simulink model "StateEstimatorForActuatorDelay"  (R2020b)
settings: Solver=FixedStepAuto  StartTime=0.0  StopTime=.5  RelTol=1e-3
values from neighbouring files (symbols this model uses):
  F = eye(6)    [MEKFAttitudeOnly.m]
  Moments = [0; 0; 0]    [Forces_and_Moments_Calculator.m]
  q = x(13:16)    [AdaptiveLQR.m]    (also in MEKF.m = nominal_state(4:7); MEKFAttitudeOnly.m = [1 0 0 0]; MEKF_old.m = nominal_state(4:7); NonlinearStateEstimationForActuatorDelay.m = x(4:7))
  r = sym('r', [3 1])    [StateSpaceController.m]    (also in TimeDelayCompensationElevator.m = [0;0]; Tracker.m = [0; 0; -(rocket_length - Average_cg)])
  ThrustTable = xlsread('F15_Thrust','Sheet1')    [ImpactVelocityNotParallelMatlab.m]    (also in OneDLanding.m; ParallelImpactVelocity.m; RunImpactVelocityParforCompiled.m)
undefined symbols (not defined in the file or in its folder): Earth, HeightAboveSeaLevel, initial_q, initial_qi, initial_w, Light, masscgI, MIL, t0, WGS84
libraries: shared6dof x4, aerolibwind2 x3, vrlib x2, shared6dofsys x2, sharedtransform x2, aerolibbdyn x1, aerolibtransform2 x1, simulink x1, sharedutil x1
settings Model: SimulationMode=accelerator  Creator=rag  LastModifiedBy=rag
settings DataIOCC: SaveFinalState=on  SaveOutput=off  SignalLogging=off  DSMLogging=off  SaveTime=off
settings OptimizationCC: DefaultParameterBehavior=Inlined  UseDivisionForNetSlopeComputation=on  GainParamInheritBuiltInType=on  UseFloatMulNetSlope=on  InlineInvariantSignals=on  EfficientFloat2IntCast=on  LifeSpan=1
settings HardwareCC: ProdLongLongMode=on
settings SFSimCC: MATLABDynamicMemAlloc=off
settings RTWCC: GenerateReport=on  LaunchReport=on
settings CodeAppCC: ForceParamTrailComments=on
settings GRTTargetCC: CombineSignalStateStructs=on  MatFileLogging=off  SupportVariableSizeSignals=on

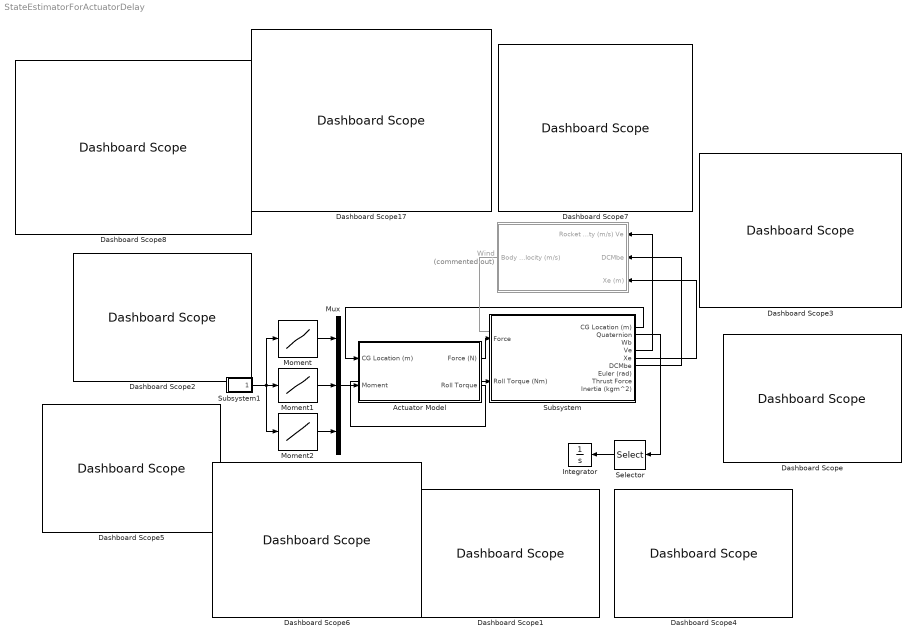
== system StateEstimatorForActuatorDelay ==
  Actuator Model : Subsystem
  Dashboard Scope{,1..8,17} (10 alike) : DashboardScope
  Integrator : Integrator  InitialCondition=initial_qi
  Moment : Lookup_n-D  NumberOfTableDimensions=1  BreakpointsForDimension1=Moments(:,1)  BreakpointsForDimension2=Moments(:,1)  BreakpointsForDimension3=Moments(:,1)  BreakpointsForDimension1FirstPoint=0  BreakpointsForDimension1Spacing=1.5e-5  Table=Moments(:,2)  ExtrapMethod=Clip  InternalRulePriority=Speed  RndMeth=Simplest  InputSameDT=on
  Moment1 : Lookup_n-D  NumberOfTableDimensions=1  BreakpointsForDimension1=Moments(:,1)  BreakpointsForDimension2=Moments(:,1)  BreakpointsForDimension3=Moments(:,1)  BreakpointsForDimension1FirstPoint=0  BreakpointsForDimension1Spacing=1.5e-5  Table=Moments(:,3)  ExtrapMethod=Clip  InternalRulePriority=Speed  RndMeth=Simplest  InputSameDT=on
  Moment2 : Lookup_n-D  NumberOfTableDimensions=1  BreakpointsForDimension1=Moments(:,1)  BreakpointsForDimension2=Moments(:,1)  BreakpointsForDimension3=Moments(:,1)  BreakpointsForDimension1FirstPoint=0  BreakpointsForDimension1Spacing=1.5e-5  Table=Moments(:,4)  ExtrapMethod=Clip  InternalRulePriority=Speed  RndMeth=Simplest  InputSameDT=on
  Mux : Mux  Inputs=3
  Selector : Selector  InputPortWidth=4  IndexOptions=Index vector (dialog)  Indices=[2:4]  OutputSizes=1
  Subsystem : Subsystem
  Subsystem1 : Subsystem
  Wind : Subsystem  Commented=on
  wires:
  Subsystem/1(CG Location (m)) -> Actuator Model/1(CG Location (m))
  Wind/1(Body Wind Velocity (m/s)) -> ?
  Actuator Model/1(Force (N)) -> Subsystem/1(Force)
  Actuator Model/2(Roll Torque) -> Subsystem/2(Roll Torque (Nm))
  Subsystem/4(Ve) -> Wind/1(Rocket velocity (m/s) Ve)
  Subsystem/6(DCMbe) -> Wind/2(DCMbe)
  Subsystem/5(Xe) -> Wind/3(Xe (m))
  Selector/1 -> Integrator/1
  Subsystem/2(Quaternion) -> Selector/1
  Moment/1 -> Mux/1
  Mux/1 -> Actuator Model/2(Moment)
  Moment1/1 -> Mux/2
  Moment2/1 -> Mux/3
  Subsystem1/1(time) -> Moment2/1, Moment/1, Moment1/1

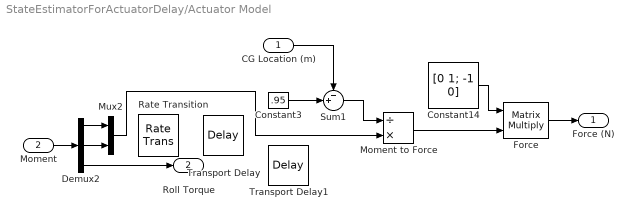
== system StateEstimatorForActuatorDelay/Actuator Model ==
  CG Location (m) : Inport
  Moment : Inport  Port=2
  Constant14 : Constant  Value=[0 1; -1 0]
  Constant3 : Constant  Value=.95
  Demux2 : Demux  Outputs=3
  Force : Product  Multiplication=Matrix(*)
  Moment to Force : Product  Inputs=/*
  Mux2 : Mux  Inputs=2
  Rate Transition : RateTransition  OutPortSampleTime=0.02
  Sum1 : Sum  Inputs=-+|
  Transport Delay : TransportDelay  DelayTime=0.07  TransDelayFeedthrough=on
  Transport Delay1 : TransportDelay  DelayTime=0.01  TransDelayFeedthrough=on
  Force (N) : Outport
  Roll Torque : Outport  Port=2
  wires:
  Demux2/1 -> Mux2/1
  Mux2/1 -> Moment to Force/2
  Sum1/1 -> Moment to Force/1
  Moment to Force/1 -> Force/2
  Constant3/1 -> Sum1/2
  Demux2/2 -> Mux2/2
  Moment/1 -> Demux2/1
  Constant14/1 -> Force/1
  Demux2/3 -> Roll Torque/1
  CG Location (m)/1 -> Sum1/1
  Force/1 -> Force (N)/1

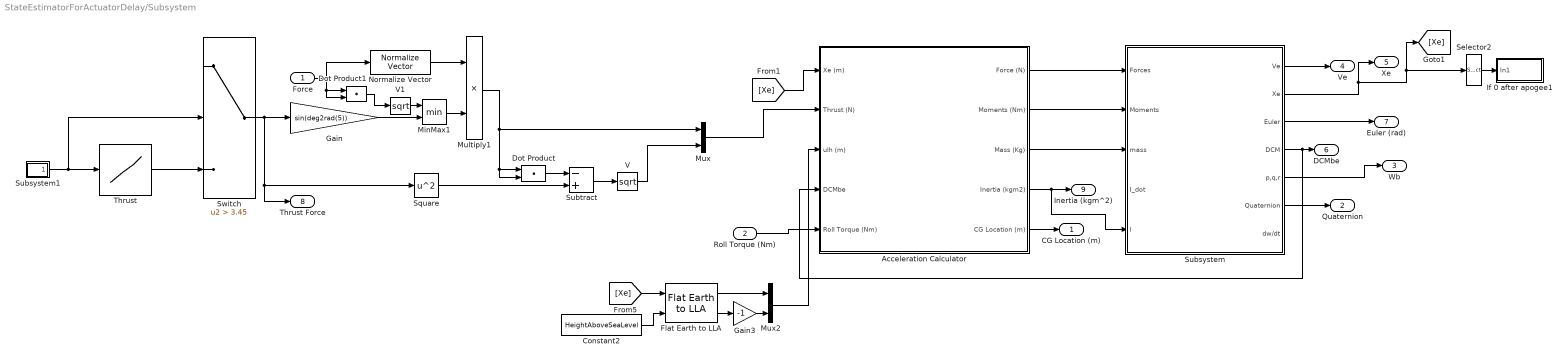
== system StateEstimatorForActuatorDelay/Subsystem ==
  Force : Inport  PortDimensions=2
  Roll Torque (Nm) : Inport  Port=2
  Acceleration Calculator : Subsystem
  Constant2 : Constant  Value=HeightAboveSeaLevel
  Dot Product : DotProduct  SaturateOnIntegerOverflow=on  OutDataTypeStr=Inherit: Inherit via internal rule
  Dot Product1 : DotProduct  SaturateOnIntegerOverflow=on  OutDataTypeStr=Inherit: Inherit via internal rule
  Flat Earth to LLA : aerolibtransform2/Flat Earth to LLA  units=Metric (MKS)  ptype=Earth (WGS84)  F=1/298.257223563  R=6378137  refPosPort=off  LL0=[21.318358277648 -157.9232805920725]  psi=0
  Gain : Gain  Gain=sin(deg2rad(5))
  Gain3 : Gain  Gain=-1
  If 0 after apogee1 : Subsystem
  MinMax1 : MinMax  Inputs=2
  Multiply1 : Product  Inputs=**
  Mux : Mux  Inputs=2
  Mux2 : Mux  Inputs=2
  Normalize Vector : vrlib/Utilities/Normalize Vector  maxzero=0
  Selector2 : Selector  InputPortWidth=3  IndexOptions=Index vector (dialog)  Indices=[3]  OutputSizes=1
  Square : Math  Operator=square  SignedPower=on  SaturateOnIntegerOverflow=on
  Subsystem : Subsystem
  Subsystem1 : Subsystem
  Subtract : Sum  Inputs=-+
  Switch : Switch  Criteria=u2 > Threshold  Threshold=3.45
  Thrust : Lookup_n-D  NumberOfTableDimensions=1  BreakpointsForDimension1=ThrustTable(:,1)  BreakpointsForDimension1FirstPoint=0  BreakpointsForDimension1Spacing=1.5e-5  Table=ThrustTable(:,2)  ExtrapMethod=Clip  InternalRulePriority=Speed  RndMeth=Simplest  InputSameDT=on
  V : Math  Operator=sqrt  SignedPower=on  SaturateOnIntegerOverflow=on
  V1 : Math  Operator=sqrt  SignedPower=on  SaturateOnIntegerOverflow=on
  CG Location (m) : Outport  VectorParamsAs1DForOutWhenUnconnected=off
  Quaternion : Outport  Port=2  VectorParamsAs1DForOutWhenUnconnected=off
  Wb : Outport  Port=3  VectorParamsAs1DForOutWhenUnconnected=off
  Ve : Outport  Port=4  VectorParamsAs1DForOutWhenUnconnected=off
  Xe : Outport  Port=5  VectorParamsAs1DForOutWhenUnconnected=off
  DCMbe : Outport  Port=6  VectorParamsAs1DForOutWhenUnconnected=off
  Euler (rad) : Outport  Port=7  VectorParamsAs1DForOutWhenUnconnected=off
  Thrust Force : Outport  Port=8  VectorParamsAs1DForOutWhenUnconnected=off
  Inertia (kgm^2) : Outport  Port=9  VectorParamsAs1DForOutWhenUnconnected=off
  wires:
  Flat Earth to LLA/1 -> Mux2/1
  Flat Earth to LLA/2 -> Gain3/1
  Gain3/1 -> Mux2/2
  Mux2/1 -> Acceleration Calculator/3(ulh (m))
  Constant2/1 -> Flat Earth to LLA/2
  [Xe] -> Acceleration Calculator/1(Xe (m))
  Selector2/1 -> If 0 after apogee1/1(In1)
  [Xe] -> Flat Earth to LLA/1
  Acceleration Calculator/5(CG Location (m)) -> CG Location (m)/1
  Acceleration Calculator/4(Inertia (kgm2)) -> Subsystem/5(I), Inertia (kgm^2)/1
  Acceleration Calculator/1(Force (N)) -> Subsystem/1(Forces)
  Acceleration Calculator/3(Mass (Kg)) -> Subsystem/3(mass)
  Mux/1 -> Acceleration Calculator/2(Thrust (N))
  Roll Torque (Nm)/1 -> Acceleration Calculator/5(Roll Torque (Nm))
  Gain/1 -> MinMax1/2
  Switch/1 -> Thrust Force/1, Square/1, Gain/1
  Subsystem1/1(time) -> Switch/2, Thrust/1
  Subsystem/1(Ve) -> Ve/1
  Subsystem/2(Xe) -> Xe/1, Selector2/1, [Xe]
  Subsystem/5(p,q,r) -> Wb/1
  Subsystem/3(Euler) -> Euler (rad)/1
  Square/1 -> Subtract/2
  Dot Product/1 -> Subtract/1
  V/1 -> Mux/2
  Subtract/1 -> V/1
  Dot Product1/1 -> V1/1
  MinMax1/1 -> Multiply1/2
  Normalize Vector/1 -> Multiply1/1
  V1/1 -> MinMax1/1
  Force/1 -> Normalize Vector/1, Dot Product1/1, Dot Product1/2
  Subsystem/6(Quaternion) -> Quaternion/1
  Subsystem/4(DCM) -> Acceleration Calculator/4(DCMbe), DCMbe/1
  Thrust/1 -> Switch/3
  Acceleration Calculator/2(Moments (Nm)) -> Subsystem/2(Moments)
  Multiply1/1 -> Mux/1, Dot Product/2, Dot Product/1

== system StateEstimatorForActuatorDelay/Subsystem1 ==
  Clock : Clock
      settings: Decimation=100
  Constant : Constant  Value=t0
  Sum : Sum  Inputs=|++
  time : Outport
  wires:
  Clock/1 -> Sum/1
  Sum/1 -> time/1
  Constant/1 -> Sum/2

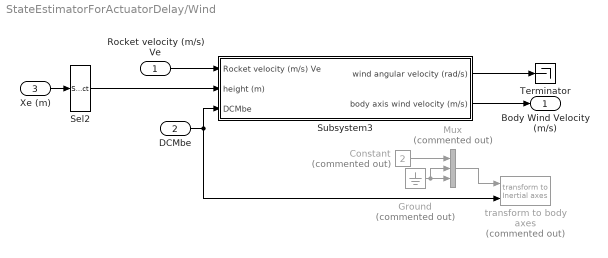
== system StateEstimatorForActuatorDelay/Wind ==
  Rocket velocity (m/s) Ve : Inport
  DCMbe : Inport  Port=2
  Xe (m) : Inport  Port=3
  Constant : Constant  Commented=on  Value=2
  Ground : Ground  Commented=on
  Mux : Mux  Commented=on  Inputs=3
  Sel2 : Selector  InputPortWidth=3  IndexOptions=Index vector (dialog)  Indices=3  OutputSizes=1
  Subsystem3 : Subsystem
  Terminator : Terminator
  transform to body axes : shared6dof/6DOF (Euler Angles)/transform to Inertial axes   Commented=on  SystemSampleTime=-1  VariantActivationTime=update diagram  Latency=0  AutoFrameSizeCalculation=off
      settings: SourceProductBaseCode=AE,PW,MT,UV,VE,VP
  Body Wind Velocity (m/s) : Outport  VectorParamsAs1DForOutWhenUnconnected=off
  wires:
  DCMbe/1 -> Subsystem3/3(DCMbe), transform to body axes/2
  Rocket velocity (m/s) Ve/1 -> Subsystem3/1(Rocket velocity (m/s) Ve)
  Mux/1 -> transform to body axes/1
  Xe (m)/1 -> Sel2/1
  Constant/1 -> Mux/1
  Subsystem3/1(wind angular velocity (rad/s)) -> Terminator/1
  Sel2/1 -> Subsystem3/2(height (m))
  Ground/1 -> Mux/2, Mux/3
  Subsystem3/2(body axis wind velocity (m/s)) -> Body Wind Velocity (m/s)/1

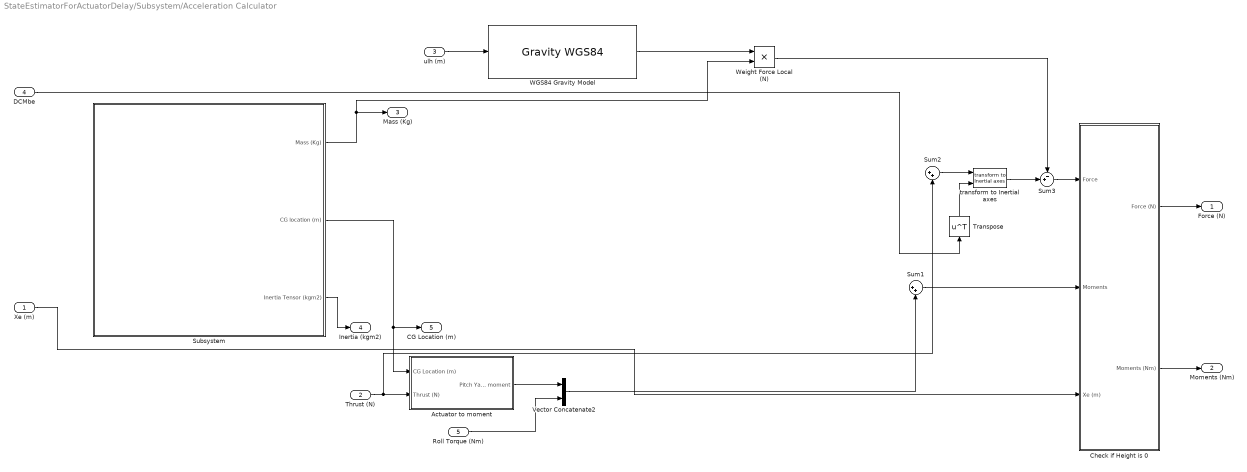
== system StateEstimatorForActuatorDelay/Subsystem/Acceleration Calculator ==
  Xe (m) : Inport
  Thrust (N) : Inport  Port=2
  ulh (m) : Inport  Port=3  PortDimensions=3
  DCMbe : Inport  Port=4
  Roll Torque (Nm) : Inport  Port=5
  Actuator to moment : Subsystem
  Check if Height is 0 : Subsystem
  Subsystem : Subsystem
  Sum1 : Sum  Inputs=|++
  Sum2 : Sum  Inputs=|++
  Sum3 : Sum  Inputs=-+|
  Transpose : Math  Operator=transpose  SignedPower=on  SaturateOnIntegerOverflow=on
  Vector Concatenate2 : Concatenate
  "WGS84 Gravity Model  " : GravityWGS84
  Weight Force Local (N) : Product
  "transform to Inertial axes " : shared6dof/6DOF (Euler Angles)/transform to Inertial axes   SystemSampleTime=-1  VariantActivationTime=update diagram  Latency=0  AutoFrameSizeCalculation=off
      settings: SourceProductBaseCode=AE,PW,MT,UV,VE,VP
  Force (N) : Outport  VectorParamsAs1DForOutWhenUnconnected=off
  Moments (Nm) : Outport  Port=2  VectorParamsAs1DForOutWhenUnconnected=off
  Mass (Kg) : Outport  Port=3  VectorParamsAs1DForOutWhenUnconnected=off
  Inertia (kgm2) : Outport  Port=4  VectorParamsAs1DForOutWhenUnconnected=off
  CG Location (m) : Outport  Port=5  VectorParamsAs1DForOutWhenUnconnected=off
  wires:
  Subsystem/3(Inertia Tensor (kgm2)) -> Inertia (kgm2)/1
  Subsystem/1(Mass (Kg)) -> Weight Force Local (N)/2, Mass (Kg)/1
  DCMbe/1 -> Transpose/1
  ulh (m)/1 -> "WGS84 Gravity Model  "/1
  Roll Torque (Nm)/1 -> Vector Concatenate2/2
  Thrust (N)/1 -> Sum2/2, Actuator to moment/2(Thrust (N))
  Actuator to moment/1(Pitch Yaw moment) -> Vector Concatenate2/1
  Xe (m)/1 -> Check if Height is 0/3(Xe (m))
  Subsystem/2(CG location (m)) -> Actuator to moment/1(CG Location (m)), CG Location (m)/1
  Weight Force Local (N)/1 -> Sum3/1
  Vector Concatenate2/1 -> Sum1/2
  Sum1/1 -> Check if Height is 0/2(Moments)
  Sum2/1 -> "transform to Inertial axes "/1
  Check if Height is 0/1(Force (N)) -> Force (N)/1
  Check if Height is 0/2(Moments (Nm)) -> Moments (Nm)/1
  "WGS84 Gravity Model  "/1 -> Weight Force Local (N)/1
  Transpose/1 -> "transform to Inertial axes "/2
  "transform to Inertial axes "/1 -> Sum3/2
  Sum3/1 -> Check if Height is 0/1(Force)

== system StateEstimatorForActuatorDelay/Subsystem/If 0 after apogee1 ==
  In1 : Inport
  Compare To Zero1 : simulink/Logic and Bit Operations/Compare To Zero  relop=<=  OutDataTypeStr=boolean
  Constant3 : Constant  Value=0.5
  Logical Operator1 : Logic  AllPortsSameDT=off  OutDataTypeStr=boolean
  Relational Operator1 : RelationalOperator  Operator=>  OutDataTypeStr=boolean  RndMeth=Simplest
  Stop Simulation1 : Stop
  Subsystem1 : Subsystem
  wires:
  Constant3/1 -> Relational Operator1/2
  In1/1 -> Compare To Zero1/1
  Logical Operator1/1 -> Stop Simulation1/1
  Compare To Zero1/1 -> Logical Operator1/2
  Relational Operator1/1 -> Logical Operator1/1
  Subsystem1/1(time) -> Relational Operator1/1

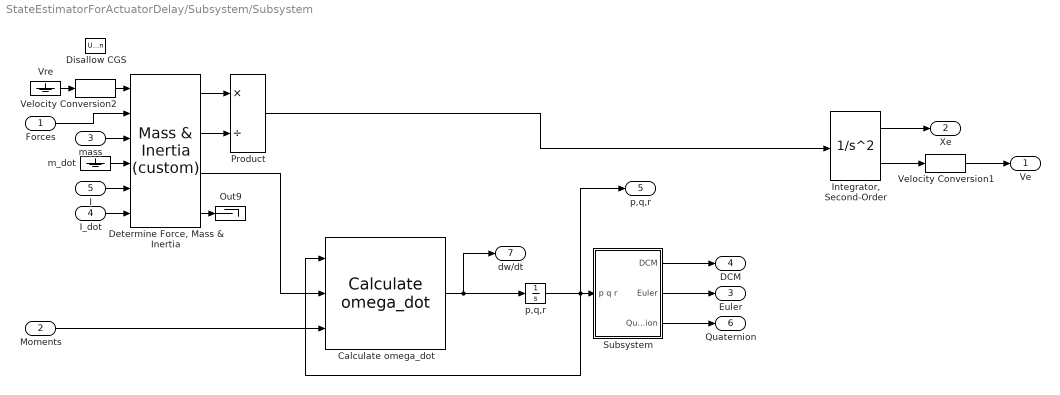
== system StateEstimatorForActuatorDelay/Subsystem/Subsystem ==
  Forces : Inport  Unit=N  PortDimensions=3
  Moments : Inport  Port=2  Unit=N*m  PortDimensions=3
  mass : Inport  Port=3  Unit=kg
  I_dot : Inport  Port=4  Unit=kg*m^2/s  PortDimensions=[3 3]
  I : Inport  Port=5  Unit=kg*m^2  PortDimensions=[3 3]
  Calculate omega_dot : shared6dofsys/Calculate omega_dot  aMode=aMode
      settings: SourceProductBaseCode=AE,PW,MT,UV,VE,VP
  "Determine Force, Mass & Inertia" : shared6dofsys/Mass & Inertia (custom)  aMode=aMode
      settings: SourceProductBaseCode=AE,PW,MT,UV,VE,VP
  Disallow CGS : UnitConfiguration  UnitSystemsStr=English,SI,SI (extended)  AllowAllUnitSystems=off
  "Integrator, Second-Order" : SecondOrderIntegrator  ICX=initial_x  LimitX=on  LowerLimitX=[-inf -inf 0]  ICDXDT=initial_v
  Out9 : Terminator
  Product : Product  Inputs=*/  SaturateOnIntegerOverflow=on  OutDataTypeStr=Inherit: Same as first input
  Subsystem : Subsystem
  Velocity Conversion1 : shared6dof/6DOF (Euler Angles)/Velocity Conversion1  SystemSampleTime=-1  VariantActivationTime=update diagram  Latency=0  AutoFrameSizeCalculation=off
      settings: SourceProductBaseCode=AE,PW,MT,UV,VE,VP
  Velocity Conversion2 : shared6dof/6DOF (Euler Angles)/Velocity Conversion2  SystemSampleTime=-1  VariantActivationTime=update diagram  Latency=0  AutoFrameSizeCalculation=off
      settings: SourceProductBaseCode=AE,PW,MT,UV,VE,VP
  Vre : Ground
  m_dot : Ground
  "p,q,r " : Integrator  InitialCondition=initial_w
  Ve : Outport  Unit=m/s  VectorParamsAs1DForOutWhenUnconnected=off
  Xe : Outport  Port=2  Unit=m  VectorParamsAs1DForOutWhenUnconnected=off
  Euler : Outport  Port=3  Unit=rad  VectorParamsAs1DForOutWhenUnconnected=off
  DCM : Outport  Port=4  Unit=1  VectorParamsAs1DForOutWhenUnconnected=off
  p,q,r : Outport  Port=5  Unit=rad/s  VectorParamsAs1DForOutWhenUnconnected=off
  Quaternion : Outport  Port=6  VectorParamsAs1DForOutWhenUnconnected=off
  dw/dt : Outport  Port=7  VectorParamsAs1DForOutWhenUnconnected=off
  wires:
  Subsystem/2(Euler) -> Euler/1
  "Determine Force, Mass & Inertia"/3 -> Calculate omega_dot/2
  "p,q,r "/1 -> Subsystem/1(p q r), p,q,r/1, Calculate omega_dot/1
  Product/1 -> "Integrator, Second-Order"/1
  mass/1 -> "Determine Force, Mass & Inertia"/3
  Velocity Conversion1/1 -> Ve/1
  Subsystem/1(DCM) -> DCM/1
  Calculate omega_dot/1 -> dw/dt/1, "p,q,r "/1
  Forces/1 -> "Determine Force, Mass & Inertia"/2
  "Determine Force, Mass & Inertia"/4 -> Out9/1
  I_dot/1 -> "Determine Force, Mass & Inertia"/6
  I/1 -> "Determine Force, Mass & Inertia"/5
  Velocity Conversion2/1 -> "Determine Force, Mass & Inertia"/1
  Vre/1 -> Velocity Conversion2/1
  "Determine Force, Mass & Inertia"/1 -> Product/1
  "Determine Force, Mass & Inertia"/2 -> Product/2
  m_dot/1 -> "Determine Force, Mass & Inertia"/4
  Subsystem/3(Quaternion) -> Quaternion/1
  "Integrator, Second-Order"/2 -> Velocity Conversion1/1
  "Integrator, Second-Order"/1 -> Xe/1
  Moments/1 -> Calculate omega_dot/3

== system StateEstimatorForActuatorDelay/Subsystem/Subsystem1 ==
  Clock : Clock
      settings: Decimation=100
  Constant : Constant  Value=t0
  Sum : Sum  Inputs=|++
  time : Outport
  wires:
  Clock/1 -> Sum/1
  Sum/1 -> time/1
  Constant/1 -> Sum/2

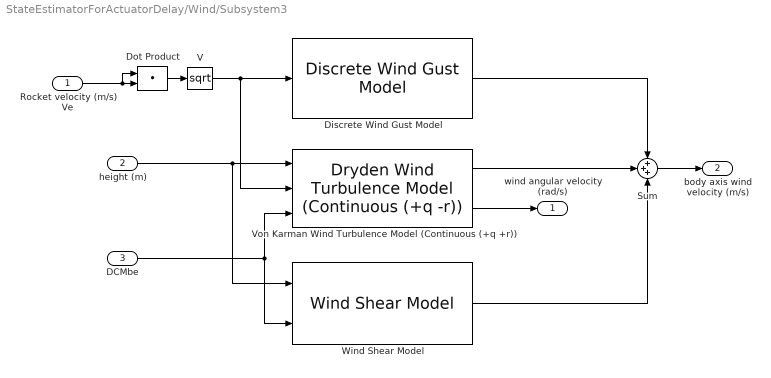
== system StateEstimatorForActuatorDelay/Wind/Subsystem3 ==
  Rocket velocity (m/s) Ve : Inport
  height (m) : Inport  Port=2
  DCMbe : Inport  Port=3
  Discrete Wind Gust Model : aerolibwind2/Discrete Wind Gust Model  units=Metric (MKS)  Gx=on  Gy=on  Gz=on  t_0=GustStart  d_m=GustLength  v_m=GuestAmplitude
  Dot Product : DotProduct  SaturateOnIntegerOverflow=on  OutDataTypeStr=Inherit: Inherit via internal rule
  Sum : Sum  Inputs=3
  V : Math  Operator=sqrt  SignedPower=on  SaturateOnIntegerOverflow=on
  Von Karman Wind Turbulence Model (Continuous (+q +r)) : aerolibwind2/Dryden Wind Turbulence Model  (Continuous (+q -r))  units=Metric (MKS)  spec=MIL-F-8785C  model=Discrete Dryden (+q -r)  W20=ShearSpeed  Wdeg=ShearDirection  TurbProb=10^-2 - Light  L_high=762  Wingspan=1  ts=0.1  Seed=[23341 23342 23343 23344]  T_on=on
  Wind Shear Model : aerolibwind2/Wind Shear Model  units=Metric (MKS)  phase=Category C - Terminal Flight Phase  W_20=ShearSpeed  Wdeg=ShearDirection
  wind angular velocity (rad/s) : Outport  VectorParamsAs1DForOutWhenUnconnected=off
  body axis wind velocity (m/s) : Outport  Port=2  VectorParamsAs1DForOutWhenUnconnected=off
  wires:
  height (m)/1 -> Wind Shear Model/1, Von Karman Wind Turbulence Model (Continuous (+q +r))/1
  Discrete Wind Gust Model/1 -> Sum/1
  DCMbe/1 -> Wind Shear Model/2, Von Karman Wind Turbulence Model (Continuous (+q +r))/3
  V/1 -> Von Karman Wind Turbulence Model (Continuous (+q +r))/2, Discrete Wind Gust Model/1
  Sum/1 -> body axis wind velocity (m/s)/1
  Wind Shear Model/1 -> Sum/3
  Von Karman Wind Turbulence Model (Continuous (+q +r))/1 -> Sum/2
  Von Karman Wind Turbulence Model (Continuous (+q +r))/2 -> wind angular velocity (rad/s)/1
  Dot Product/1 -> V/1
  Rocket velocity (m/s) Ve/1 -> Dot Product/1, Dot Product/2

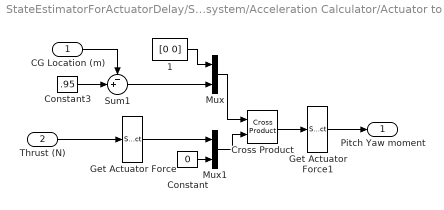
== system StateEstimatorForActuatorDelay/Subsystem/Acceleration Calculator/Actuator to moment ==
  CG Location (m) : Inport
  Thrust (N) : Inport  Port=2
  1 : Constant  Value=[0 0]
  Constant : Constant  Value=0
  Constant3 : Constant  Value=.95
  Cross Product : vrlib/Utilities/Cross Product
  Get Actuator Force : Selector  InputPortWidth=3  IndexOptions=Index vector (dialog)  Indices=[1 2]  OutputSizes=1
  Get Actuator Force1 : Selector  InputPortWidth=3  IndexOptions=Index vector (dialog)  Indices=[1 2]  OutputSizes=1
  Mux : Mux  Inputs=2
  Mux1 : Mux  Inputs=2
  Sum1 : Sum  Inputs=-+|
  Pitch Yaw moment : Outport  VectorParamsAs1DForOutWhenUnconnected=off
  wires:
  Constant3/1 -> Sum1/2
  Get Actuator Force/1 -> Mux1/1
  CG Location (m)/1 -> Sum1/1
  Thrust (N)/1 -> Get Actuator Force/1
  Cross Product/1 -> Get Actuator Force1/1
  Mux/1 -> Cross Product/1
  Sum1/1 -> Mux/2
  1/1 -> Mux/1
  Mux1/1 -> Cross Product/2
  Constant/1 -> Mux1/2
  Get Actuator Force1/1 -> Pitch Yaw moment/1

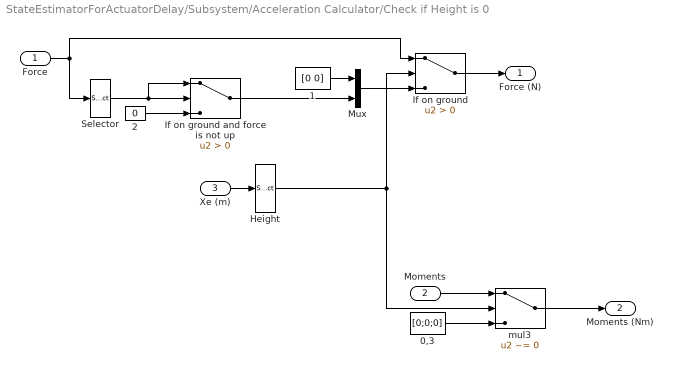
== system StateEstimatorForActuatorDelay/Subsystem/Acceleration Calculator/Check if Height is 0 ==
  Force : Inport
  Moments : Inport  Port=2
  Xe (m) : Inport  Port=3
  0,3 : Constant  Value=[0;0;0]
  1 : Constant  Value=[0 0]
  2 : Constant  Value=0
  Height : Selector  InputPortWidth=3  IndexOptions=Index vector (dialog)  Indices=3  OutputSizes=1
  If on ground : Switch  Criteria=u2 > Threshold
  If on ground and force is not up : Switch  Criteria=u2 > Threshold
  Mux : Mux  Inputs=2
  Selector : Selector  InputPortWidth=3  IndexOptions=Index vector (dialog)  Indices=3  OutputSizes=1
  mul3 : Switch  Criteria=u2 ~= 0  Threshold=deg2rad(17)
  Force (N) : Outport  VectorParamsAs1DForOutWhenUnconnected=off
  Moments (Nm) : Outport  Port=2  VectorParamsAs1DForOutWhenUnconnected=off
  wires:
  Moments/1 -> mul3/1
  Force/1 -> If on ground/1, Selector/1
  Xe (m)/1 -> Height/1
  0,3/1 -> mul3/3
  Height/1 -> If on ground/2, mul3/2
  2/1 -> If on ground and force is not up/3
  Selector/1 -> If on ground and force is not up/1, If on ground and force is not up/2
  1/1 -> Mux/1
  Mux/1 -> If on ground/3
  If on ground and force is not up/1 -> Mux/2
  If on ground/1 -> Force (N)/1
  mul3/1 -> Moments (Nm)/1

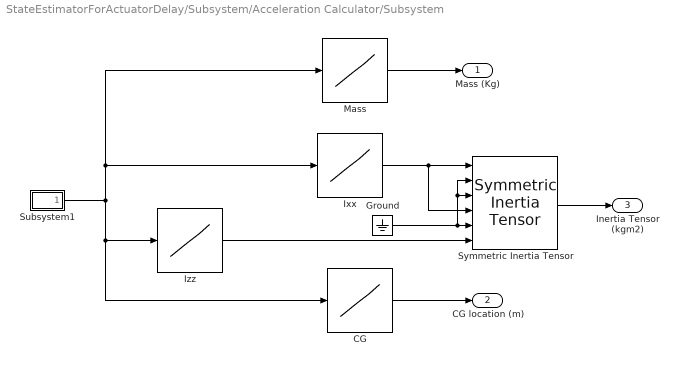
== system StateEstimatorForActuatorDelay/Subsystem/Acceleration Calculator/Subsystem ==
  CG : Lookup_n-D  NumberOfTableDimensions=1  BreakpointsForDimension1=masscgI(:,1)  BreakpointsForDimension1FirstPoint=0  BreakpointsForDimension1Spacing=1.5e-5  Table=masscgI(:,5)  ExtrapMethod=Clip  InternalRulePriority=Speed  RndMeth=Simplest  InputSameDT=on
  Ground : Ground
  Ixx : Lookup_n-D  NumberOfTableDimensions=1  BreakpointsForDimension1=masscgI(:,1)  BreakpointsForDimension1FirstPoint=0  BreakpointsForDimension1Spacing=1.5e-5  Table=masscgI(:,3)  ExtrapMethod=Clip  InternalRulePriority=Speed  RndMeth=Simplest  InputSameDT=on
  Izz : Lookup_n-D  NumberOfTableDimensions=1  BreakpointsForDimension1=masscgI(:,1)  BreakpointsForDimension1FirstPoint=0  BreakpointsForDimension1Spacing=1.5e-5  Table=masscgI(:,4)  ExtrapMethod=Clip  InternalRulePriority=Speed  RndMeth=Simplest  InputSameDT=on
  Mass : Lookup_n-D  NumberOfTableDimensions=1  BreakpointsForDimension1=masscgI(:,1)  BreakpointsForDimension1FirstPoint=0  BreakpointsForDimension1Spacing=1.5e-5  Table=masscgI(:,2)  ExtrapMethod=Clip  InternalRulePriority=Speed  RndMeth=Simplest  InputSameDT=on
  Subsystem1 : Subsystem
  Symmetric Inertia Tensor : aerolibbdyn/Symmetric Inertia Tensor
      settings: SourceProductBaseCode=AE
  Mass (Kg) : Outport  VectorParamsAs1DForOutWhenUnconnected=off
  CG location (m) : Outport  Port=2  VectorParamsAs1DForOutWhenUnconnected=off
  Inertia Tensor (kgm2) : Outport  Port=3  VectorParamsAs1DForOutWhenUnconnected=off
  wires:
  Ground/1 -> Symmetric Inertia Tensor/2, Symmetric Inertia Tensor/3, Symmetric Inertia Tensor/5
  Symmetric Inertia Tensor/1 -> Inertia Tensor (kgm2)/1
  Subsystem1/1(time) -> Izz/1, CG/1, Ixx/1, Mass/1
  Mass/1 -> Mass (Kg)/1
  Ixx/1 -> Symmetric Inertia Tensor/4, Symmetric Inertia Tensor/1
  Izz/1 -> Symmetric Inertia Tensor/6
  CG/1 -> CG location (m)/1

== system StateEstimatorForActuatorDelay/Subsystem/If 0 after apogee1/Subsystem1 ==
  Clock : Clock
      settings: Decimation=100
  Constant : Constant  Value=t0
  Sum : Sum  Inputs=|++
  time : Outport
  wires:
  Clock/1 -> Sum/1
  Sum/1 -> time/1
  Constant/1 -> Sum/2

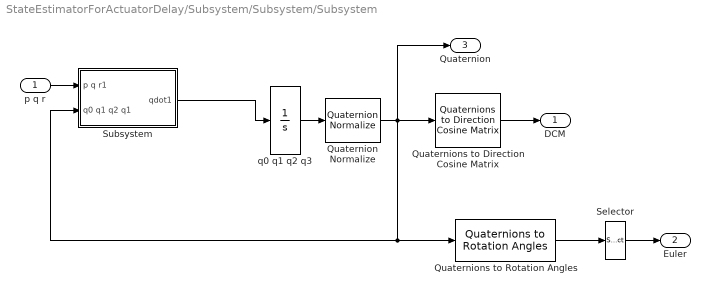
== system StateEstimatorForActuatorDelay/Subsystem/Subsystem/Subsystem ==
  p q r : Inport
  Quaternion Normalize : sharedutil/Quaternion Normalize  aMode=aMode
      settings: SourceProductBaseCode=AE,PW,MT,UV,VE,VP
  Quaternions to Direction Cosine Matrix : sharedtransform/Quaternions to  Direction Cosine Matrix  aMode=aMode
      settings: SourceProductBaseCode=AE,PW,MT,UV,VE,VP
  Quaternions to Rotation Angles : sharedtransform/Quaternions to Rotation Angles  rotationOrder=ZYX  aMode=aMode
      settings: SourceProductBaseCode=AE,PW,MT,UV,VE,VP
  Selector : Selector  IndexMode=Zero-based  InputPortWidth=3  IndexOptions=Index vector (dialog)  Indices=[ 2 1 0]  OutputSizes=1
  Subsystem : Subsystem
  q0 q1 q2 q3 : Integrator  InitialCondition=initial_q
  DCM : Outport  VectorParamsAs1DForOutWhenUnconnected=off
  Euler : Outport  Port=2  VectorParamsAs1DForOutWhenUnconnected=off
  Quaternion : Outport  Port=3  VectorParamsAs1DForOutWhenUnconnected=off
  wires:
  Selector/1 -> Euler/1
  q0 q1 q2 q3/1 -> Quaternion Normalize/1
  Quaternions to Direction Cosine Matrix/1 -> DCM/1
  Subsystem/1(qdot1) -> q0 q1 q2 q3/1
  p q r/1 -> Subsystem/1(p q r1)
  Quaternions to Rotation Angles/1 -> Selector/1
  Quaternion Normalize/1 -> Quaternion/1, Subsystem/2(q0 q1 q2 q1), Quaternions to Rotation Angles/1, Quaternions to Direction Cosine Matrix/1

== system StateEstimatorForActuatorDelay/Subsystem/Acceleration Calculator/Subsystem/Subsystem1 ==
  Clock : Clock
      settings: Decimation=100
  Constant : Constant  Value=t0
  Sum : Sum  Inputs=|++
  time : Outport
  wires:
  Clock/1 -> Sum/1
  Sum/1 -> time/1
  Constant/1 -> Sum/2

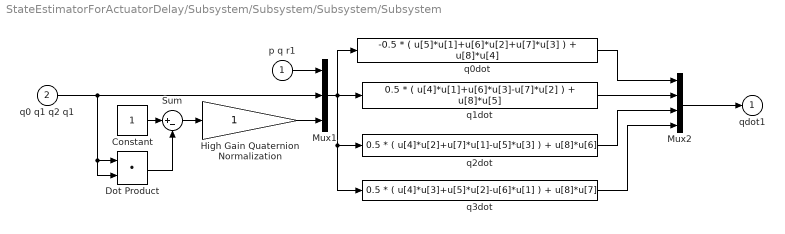
== system StateEstimatorForActuatorDelay/Subsystem/Subsystem/Subsystem/Subsystem ==
  p q r1 : Inport
  q0 q1 q2 q1 : Inport  Port=2
  Constant : Constant
  Dot Product : DotProduct  OutDataTypeStr=Inherit: Inherit via internal rule
  High Gain Quaternion Normalization : Gain  SaturateOnIntegerOverflow=on  OutDataTypeStr=Inherit: Same as input  ParamDataTypeStr=Inherit: Same as input
  Mux1 : Mux  Inputs=[3 4 1]
  Mux2 : Mux
  Sum : Sum  Inputs=|+-  InputSameDT=on  SaturateOnIntegerOverflow=on  OutDataTypeStr=Inherit: Same as first input
  q0dot : Fcn  Expr=-0.5 * ( u[5]*u[1]+u[6]*u[2]+u[7]*u[3] ) + u[8]*u[4]
  q1dot : Fcn  Expr=0.5 * ( u[4]*u[1]+u[6]*u[3]-u[7]*u[2] ) + u[8]*u[5]
  q2dot : Fcn  Expr=0.5 * ( u[4]*u[2]+u[7]*u[1]-u[5]*u[3] ) + u[8]*u[6]
  q3dot : Fcn  Expr=0.5 * ( u[4]*u[3]+u[5]*u[2]-u[6]*u[1] ) + u[8]*u[7]
  qdot1 : Outport  InitialOutput=0  VectorParamsAs1DForOutWhenUnconnected=off
  wires:
  Constant/1 -> Sum/1
  Dot Product/1 -> Sum/2
  Mux1/1 -> q2dot/1, q3dot/1, q0dot/1, q1dot/1
  q0 q1 q2 q1/1 -> Dot Product/1, Dot Product/2, Mux1/2
  Sum/1 -> High Gain Quaternion Normalization/1
  Mux2/1 -> qdot1/1
  q0dot/1 -> Mux2/1
  q3dot/1 -> Mux2/4
  q1dot/1 -> Mux2/2
  q2dot/1 -> Mux2/3
  High Gain Quaternion Normalization/1 -> Mux1/3
  p q r1/1 -> Mux1/1
